simulink library "fixedGroundStation_cl"  (R2018b)
settings: Solver=VariableStepAuto  StartTime=0.0  StopTime=10.0  RelTol=1e-3
undefined symbols (not defined in the file or in its folder): gndStnMmtArms, ini_platform_ang, ini_platform_vel, sim_param
libraries: simulink x1, eulAng2RotMat_ul x1, massSpringDamper_ul x1, thrAttachPtKinematics_ul x1, tethersMoment_cl x1
settings Model: Creator=M.Cobb  LastModifiedBy=Erin B

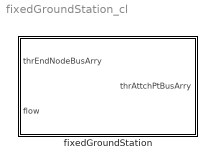
== system fixedGroundStation_cl ==
  fixedGroundStation : Subsystem  mask{fixed=1, J=sim_param.platform_param.platform_Izz, b=sim_param.platform_param.platform_damping, posVec=[0 0 0], thr1AttachPt=sim_param.tether_imp_nodes.R11_g, thr2AttachPt=sim_param.tether_imp_nodes.R21_g, thr3AttachPt=sim_param.tether_imp_nodes.R31_g, initAngPos=ini_platform_ang, initAngVel=ini_platform_vel}
      mask prompts: fixed "Free Spin Enable (==0 -> No Rotation, ~=0 -> Free Spinning)"; J "Rotational Inertia"; b "Damping coefficient"; posVec "Position Vector"; thr1AttachPt "Tether 1"; thr2AttachPt "Tether 2"; thr3AttachPt "Tether 3"; initAngPos "Initial angle"; initAngVel "Inital angular velocity"
      mask DialogControl Container5 Prompt: Physical Parameters
      mask DialogControl Container3 Prompt: Tether attachment position vectors: platform frame
      mask DialogControl Container4 Prompt: Initial conditions

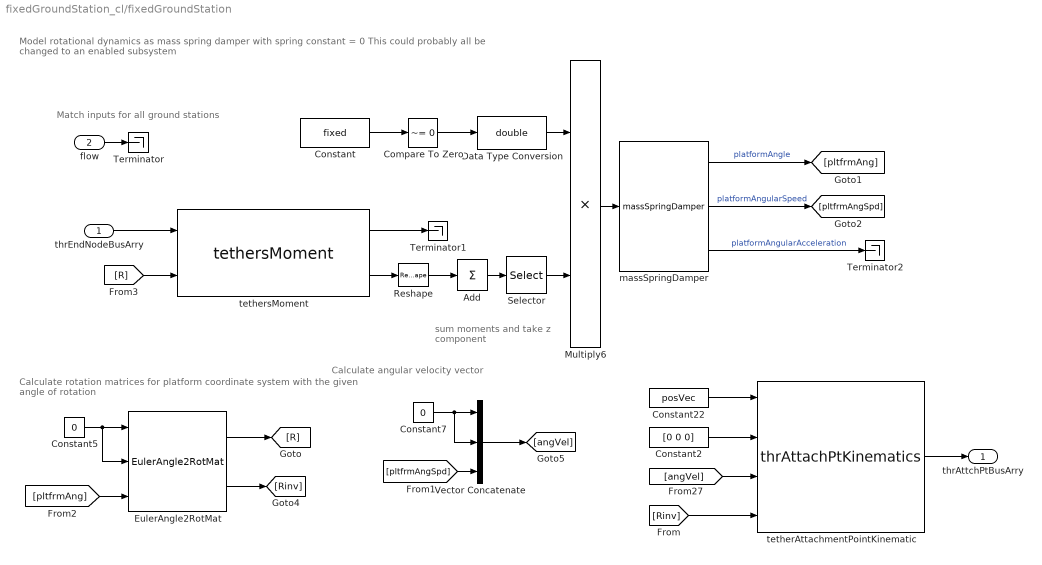
== system fixedGroundStation_cl/fixedGroundStation ==
  note: Match inputs for all ground stations
  note: sum moments and
      | take z component
  note: Calculate rotation matrices for platform coordinate
      | system with the given angle of rotation
  note: Calculate angular velocity vector
  note: Model rotational dynamics as mass spring damper with
      | spring constant = 0
      | This could probably all be changed to an enabled subsystem
  thrEndNodeBusArry : Inport
  flow : Inport  Port=2
  Add : Sum  Inputs=+  CollapseMode=Specified dimension  CollapseDim=2
  Compare To Zero : simulink/Logic and Bit Operations/Compare To Zero  relop=~=  OutDataTypeStr=boolean
  Constant : Constant  Value=fixed
  Constant2 : Constant  Value=[0 0 0]
  Constant22 : Constant  Value=posVec
  Constant5 : Constant  Value=0
  Constant7 : Constant  Value=0
  Data Type Conversion : DataTypeConversion  OutDataTypeStr=double
  EulerAngle2RotMat : eulAng2RotMat_ul/EulerAngle2RotMat  SystemSampleTime=-1
  Multiply6 : Product
  Reshape : Reshape  OutputDimensionality=Customize  OutputDimensions=[3 numel(gndStnMmtArms)]
  Selector : Selector  InputPortWidth=3  IndexOptions=Index vector (dialog)  Indices=3  OutputSizes=1
  Terminator : Terminator
  Terminator1 : Terminator
  Terminator2 : Terminator
  Vector Concatenate : Concatenate  NumInputs=3
  massSpringDamper : massSpringDamper_ul/massSpringDamper  m=J  b=b  k=0  x0=initAngPos  xDot0=initAngVel
  tetherAttachmentPointKinematic : thrAttachPtKinematics_ul/thrAttachPtKinematics  atchPts=gndStnMmtArms
  tethersMoment : tethersMoment_cl/tethersMoment  arms=gndStnMmtArms
  thrAttchPtBusArry : Outport
  wires:
  Constant5/1 -> EulerAngle2RotMat/2, EulerAngle2RotMat/1
  EulerAngle2RotMat/1 -> [R]
  EulerAngle2RotMat/2 -> [Rinv]
  Constant7/1 -> Vector Concatenate/1, Vector Concatenate/2
  Vector Concatenate/1 -> [angVel]
  massSpringDamper/2 -> [pltfrmAngSpd]  "platformAngularSpeed"
  Constant/1 -> Compare To Zero/1
  Compare To Zero/1 -> Data Type Conversion/1
  massSpringDamper/3 -> Terminator2/1  "platformAngularAcceleration"
  Multiply6/1 -> massSpringDamper/1
  Data Type Conversion/1 -> Multiply6/1
  Selector/1 -> Multiply6/2
  tetherAttachmentPointKinematic/1 -> thrAttchPtBusArry/1
  massSpringDamper/1 -> [pltfrmAng]  "platformAngle"
  thrEndNodeBusArry/1 -> tethersMoment/1
  [R] -> tethersMoment/2
  tethersMoment/2 -> Reshape/1
  Reshape/1 -> Add/1
  Add/1 -> Selector/1
  Constant22/1 -> tetherAttachmentPointKinematic/1
  Constant2/1 -> tetherAttachmentPointKinematic/2
  [Rinv] -> tetherAttachmentPointKinematic/4
  [angVel] -> tetherAttachmentPointKinematic/3
  tethersMoment/1 -> Terminator1/1
  [pltfrmAngSpd] -> Vector Concatenate/3
  [pltfrmAng] -> EulerAngle2RotMat/3
  flow/1 -> Terminator/1
